simulink model "TRAS_2dof_model"  (Simulink 10.3)
settings: Solver=ode3  StartTime=0.0  StopTime=20  FixedStep=.02  RelTol=1e-3  EnableMultiTasking=on
PreLoadFcn:
  | load tras_char
values from neighbouring files (symbols this model uses):
  control_a = [-1 -0.975 -0.95 -0.925 -0.9 -0.875 -0.85 -0.825 -0.8 -0.775 -0.75 -0.725 ... (81 elements, 1x81)]    [tras_char.mat]
  control_p = [-1 -0.975 -0.95 -0.925 -0.9 -0.875 -0.85 -0.825 -0.8 -0.775 -0.75 -0.725 ... (81 elements, 1x81)]    [tras_char.mat]
  force_a = [-0.649258706417 -0.618583933776 -0.596035206849 -0.571018846476 -0.551435310746 -0.523759715026 -0.511848182481 -0.49454126862 -0.462774567546 -0.442304535703 -0.437765206714 -0.399946095099 ... (81 elements, 1x81)]    [tras_char.mat]
  force_p = [-0.71417078206 -0.698541481137 -0.676359428972 -0.657306593399 -0.636149510201 -0.615949677515 -0.602138570677 -0.585879142379 -0.565408182885 -0.543655801355 -0.527755120628 -0.502405059235 ... (81 elements, 1x81)]    [tras_char.mat]
  rpm_a = [-6404.51002569 -6293.6960338 -6182.86749781 -6046.13242895 -5923.80032552 -5809.50701506 -5681.9476375 -5554.98805062 -5417.12878392 -5272.02245615 -5158.44672314 -5027.94718311 ... (81 elements, 1x81)]    [tras_char.mat]
  rpm_p = [-3678.29210985 -3557.9090356 -3500.75969748 -3468.48920637 -3408.40308809 -3364.59631401 -3305.24812764 -3268.16062475 -3204.9654373 -3137.29807834 -3101.82489983 -3044.64042209 ... (81 elements, 1x81)]    [tras_char.mat]
settings Model: Creator=inteco  LastModifiedBy=inteco  MultithreadedSim=on
settings DataIOCC: LimitDataPoints=on  SignalLoggingName=sigsOut
settings DebuggingCC: SaveWithParameterizedLinksMsg=none  SignalResolutionControl=TryResolveAllWithWarning  MultiTaskDSMMsg=warning  MultiTaskCondExecSysMsg=none  PregeneratedLibrarySubsystemCodeDiagnostic=none
settings HardwareCC: TargetUnknown=on
settings ConfigComp: CovSFcnEnable=off

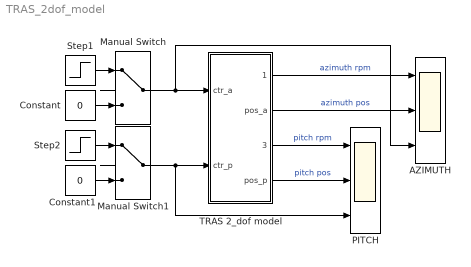
== system TRAS_2dof_model ==
  AZIMUTH : Scope  NumInputPorts=3
  Constant : Constant  Value=0
  Constant1 : Constant  Value=0
  Manual Switch : ManualSwitch
  Manual Switch1 : ManualSwitch
  PITCH : Scope  NumInputPorts=3
  Step1 : Step  SampleTime=0
  Step2 : Step  SampleTime=0
  "TRAS 2_dof model " : Subsystem
  wires:
  "TRAS 2_dof model "/1(rpm_a) -> AZIMUTH/1  "azimuth rpm"
  "TRAS 2_dof model "/2(pos_a) -> AZIMUTH/2  "azimuth pos"
  Manual Switch/1 -> "TRAS 2_dof model "/1(ctr_a), AZIMUTH/3
  Step1/1 -> Manual Switch/1
  Constant/1 -> Manual Switch/2
  Step2/1 -> Manual Switch1/1
  Constant1/1 -> Manual Switch1/2
  Manual Switch1/1 -> "TRAS 2_dof model "/2(ctr_p), PITCH/3
  "TRAS 2_dof model "/3(rpm_p) -> PITCH/1  "pitch rpm"
  "TRAS 2_dof model "/4(pos_p) -> PITCH/2  "pitch pos"

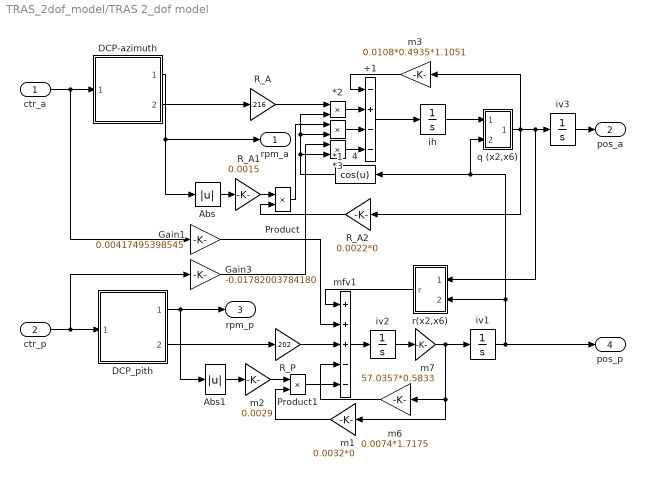
== system TRAS_2dof_model/TRAS 2_dof model  ==
  ctr_a : Inport
  ctr_p : Inport  Port=2
  *1 : Product  InputSameDT=on  SaturateOnIntegerOverflow=on  OutDataTypeStr=Inherit: Same as first input
  *2 : Product  InputSameDT=on  SaturateOnIntegerOverflow=on  OutDataTypeStr=Inherit: Same as first input
  *3 : Product  InputSameDT=on  SaturateOnIntegerOverflow=on  OutDataTypeStr=Inherit: Same as first input
  +1 : Sum  Inputs=-+--  InputSameDT=on  SaturateOnIntegerOverflow=on  OutDataTypeStr=Inherit: Same as first input
  4 : Fcn  Expr=cos(u)
  Abs : Abs  SaturateOnIntegerOverflow=on
  Abs1 : Abs  SaturateOnIntegerOverflow=on
  DCP-azimuth : Subsystem
  DCP_pith : Subsystem
  Gain1 : Gain  Gain=0.00417495398545  SaturateOnIntegerOverflow=on  OutDataTypeStr=Inherit: Same as input  ParamDataTypeStr=Inherit: Same as input
  Gain3 : Gain  Gain=-0.01782003784180  SaturateOnIntegerOverflow=on  OutDataTypeStr=Inherit: Same as input  ParamDataTypeStr=Inherit: Same as input
  Product : Product  InputSameDT=on  SaturateOnIntegerOverflow=on  OutDataTypeStr=Inherit: Same as first input
  Product1 : Product  SaturateOnIntegerOverflow=on  OutDataTypeStr=Inherit: Same as first input
  R_A : Gain  Gain=.216  OutDataTypeStr=Inherit: Same as input  ParamDataTypeStr=Inherit: Same as input
  R_A1 : Gain  Gain=0.0015  OutDataTypeStr=Inherit: Same as input  ParamDataTypeStr=Inherit: Same as input
  R_A2 : Gain  Gain=0.0022*0  OutDataTypeStr=Inherit: Same as input  ParamDataTypeStr=Inherit: Same as input
  R_P : Gain  Gain=.202  OutDataTypeStr=Inherit: Same as input  ParamDataTypeStr=Inherit: Same as input
  ih : Integrator  UpperSaturationLimit=10  LowerSaturationLimit=-10
  iv1 : Integrator  LimitOutput=on  UpperSaturationLimit=pi/2  LowerSaturationLimit=-pi/2
  iv2 : Integrator  UpperSaturationLimit=pi  LowerSaturationLimit=-pi
  iv3 : Integrator  LimitOutput=on  UpperSaturationLimit=6  LowerSaturationLimit=-6
  m1 : Gain  Gain=0.0032*0  SaturateOnIntegerOverflow=on  OutDataTypeStr=Inherit: Same as input  ParamDataTypeStr=Inherit: Same as input
  m2 : Gain  Gain=0.0029  SaturateOnIntegerOverflow=on  OutDataTypeStr=Inherit: Same as input  ParamDataTypeStr=Inherit: Same as input
  m3 : Gain  Gain=0.0108*0.4935*1.1051  OutDataTypeStr=Inherit: Same as input  ParamDataTypeStr=Inherit: Same as input
  m6 : Gain  Gain=0.0074*1.7175  OutDataTypeStr=Inherit: Same as input  ParamDataTypeStr=Inherit: Same as input
  m7 : Gain  Gain=57.0357*0.5833  SaturateOnIntegerOverflow=on  OutDataTypeStr=Inherit: Same as input  ParamDataTypeStr=Inherit: Same as input
  mfv1 : Sum  Inputs=+++--  InputSameDT=on  SaturateOnIntegerOverflow=on  OutDataTypeStr=Inherit: Same as first input
  q (x2,x6) : Subsystem
  r(x2,x6) : Subsystem
  rpm_a : Outport  VectorParamsAs1DForOutWhenUnconnected=off
  pos_a : Outport  Port=2  VectorParamsAs1DForOutWhenUnconnected=off
  rpm_p : Outport  Port=3  VectorParamsAs1DForOutWhenUnconnected=off
  pos_p : Outport  Port=4  VectorParamsAs1DForOutWhenUnconnected=off
  wires:
  DCP-azimuth/2(FORCE_A) -> R_A/1
  *1/1 -> +1/3
  m3/1 -> +1/1
  *2/1 -> +1/2
  ih/1 -> q (x2,x6)/1(x2)
  q (x2,x6)/1(q) -> iv3/1, r(x2,x6)/1(y2), m3/1, R_A2/1
  R_A/1 -> *2/1
  Abs/1 -> R_A1/1
  R_A1/1 -> Product/1
  R_A2/1 -> Product/2
  DCP_pith/2(FORCE_P) -> R_P/1
  m6/1 -> mfv1/4
  iv2/1 -> m7/1
  mfv1/1 -> iv2/1
  m7/1 -> iv1/1, m6/1, m1/1
  DCP_pith/1(RPM_P) -> Abs1/1, rpm_p/1
  Abs1/1 -> m2/1
  Product1/1 -> mfv1/5
  r(x2,x6)/1(r) -> mfv1/1
  R_P/1 -> mfv1/3
  iv1/1 -> pos_p/1, r(x2,x6)/2(x6), 4/1, q (x2,x6)/2(x6)
  m1/1 -> Product1/2
  m2/1 -> Product1/1
  *3/1 -> +1/4
  Product/1 -> *1/1
  4/1 -> *2/2, *1/2, *3/2
  Gain1/1 -> mfv1/2
  Gain3/1 -> *3/1
  ctr_a/1 -> DCP-azimuth/1(CTR_A), Gain1/1
  ctr_p/1 -> DCP_pith/1(CTR_P), Gain3/1
  iv3/1 -> pos_a/1
  +1/1 -> ih/1
  DCP-azimuth/1(RPM_A) -> rpm_a/1, Abs/1

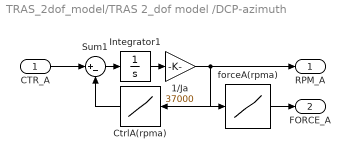
== system TRAS_2dof_model/TRAS 2_dof model /DCP-azimuth ==
  CTR_A : Inport
  1/Ja : Gain  Gain=37000  SaturateOnIntegerOverflow=on  OutDataTypeStr=Inherit: Same as input  ParamDataTypeStr=Inherit: Same as input
  CtrlA(rpma) : Lookup  InputValues=rpm_a  Table=control_a  SaturateOnIntegerOverflow=on
  Integrator1 : Integrator
  Sum1 : Sum  Inputs=|+-  InputSameDT=on  SaturateOnIntegerOverflow=on  OutDataTypeStr=Inherit: Same as first input
  forceA(rpma) : Lookup  InputValues=rpm_a  Table=force_a  SaturateOnIntegerOverflow=on
  RPM_A : Outport  VectorParamsAs1DForOutWhenUnconnected=off
  FORCE_A : Outport  Port=2  VectorParamsAs1DForOutWhenUnconnected=off
  wires:
  Sum1/1 -> Integrator1/1
  CtrlA(rpma)/1 -> Sum1/2
  Integrator1/1 -> 1/Ja/1
  1/Ja/1 -> CtrlA(rpma)/1, forceA(rpma)/1, RPM_A/1
  CTR_A/1 -> Sum1/1
  forceA(rpma)/1 -> FORCE_A/1

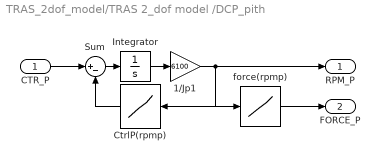
== system TRAS_2dof_model/TRAS 2_dof model /DCP_pith ==
  CTR_P : Inport
  1/Jp1 : Gain  Gain=6100  OutDataTypeStr=Inherit: Same as input  ParamDataTypeStr=Inherit: Same as input
  CtrlP(rpmp) : Lookup  InputValues=rpm_p  Table=control_p  SaturateOnIntegerOverflow=on
  Integrator : Integrator
  Sum : Sum  Inputs=|+-  InputSameDT=on  SaturateOnIntegerOverflow=on  OutDataTypeStr=Inherit: Same as first input
  force(rpmp) : Lookup  InputValues=rpm_p  Table=force_p  SaturateOnIntegerOverflow=on
  RPM_P : Outport  VectorParamsAs1DForOutWhenUnconnected=off
  FORCE_P : Outport  Port=2  VectorParamsAs1DForOutWhenUnconnected=off
  wires:
  Sum/1 -> Integrator/1
  Integrator/1 -> 1/Jp1/1
  CtrlP(rpmp)/1 -> Sum/2
  1/Jp1/1 -> CtrlP(rpmp)/1, force(rpmp)/1, RPM_P/1
  CTR_P/1 -> Sum/1
  force(rpmp)/1 -> FORCE_P/1

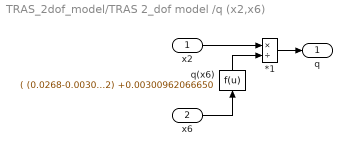
== system TRAS_2dof_model/TRAS 2_dof model /q (x2,x6) ==
  x2 : Inport
  x6 : Inport  Port=2
  " q(x6)" : Fcn  Expr=( (0.0268-0.00300962066650)*cos(u)^2) +0.00300962066650
  *1 : Product  Inputs=*/  InputSameDT=on  SaturateOnIntegerOverflow=on  OutDataTypeStr=Inherit: Same as first input
  q : Outport  VectorParamsAs1DForOutWhenUnconnected=off
  wires:
  *1/1 -> q/1
  x2/1 -> *1/1
  x6/1 -> " q(x6)"/1
  " q(x6)"/1 -> *1/2

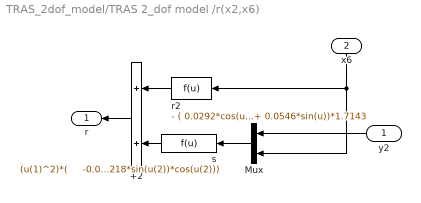
== system TRAS_2dof_model/TRAS 2_dof model /r(x2,x6) ==
  y2 : Inport
  x6 : Inport  Port=2
  +2 : Sum  InputSameDT=on  SaturateOnIntegerOverflow=on  OutDataTypeStr=Inherit: Same as first input
  Mux : Mux  Inputs=2
  r2 : Fcn  Expr=- ( 0.0292*cos(u)+ 0.0546*sin(u))*1.7143
  s : Fcn  Expr="(u(1)^2)*(     -0.07389953104162*  0.28753198180218*sin(u(2))*cos(u(2)))"
  r : Outport  VectorParamsAs1DForOutWhenUnconnected=off
  wires:
  Mux/1 -> s/1
  r2/1 -> +2/1
  s/1 -> +2/2
  x6/1 -> Mux/2, r2/1
  +2/1 -> r/1
  y2/1 -> Mux/1
